simulink model "Supine_SpeedGoat_v1_final"  (R2022a)
settings: Solver=ode5  StartTime=0.0  StopTime=Inf  FixedStep=0.001  RelTol=1e-3  EnableMultiTasking=on
undefined symbols (not defined in the file): Ended, Low, Single
libraries: speedgoatlib_IO191 x5, dsparch4 x4, dspswit3 x2, slrealtimeutilitieslib x2, slrealtimeiplib x2, dspsigops x1
settings Model: SimulationMode=external  ExtModeEnableFloating=off  Creator=sjalal6  LastModifiedBy=rbme1
settings SolverCC: ConcurrentTasks=on  AlgebraicLoopSolver=TrustRegion  PositivePriorityOrder=on
settings DataIOCC: ExternalInput=waveform  LimitDataPoints=on  LoadExternalInput=on  SaveFormat=Array  SignalLoggingSaveFormat=ModelDataLogs  ReturnWorkspaceOutputs=off
settings OptimizationCC: BlockReduction=off  OptimizeBlockIOStorage=off  BufferReuse=off  ExpressionFolding=off  ExpressionDepthLimit=2147483647  LocalBlockOutputs=off
settings DebuggingCC: UnderspecifiedInitializationDetection=Classic  MergeDetectMultiDrivingBlocksExec=none  SolverPrmCheckMsg=warning  TasksWithSamePriorityMsg=none  ParameterPrecisionLossMsg=none  FcnCallInpInsideContextMsg=warning  UnconnectedInputMsg=warning  UnconnectedOutputMsg=warning  UnconnectedLineMsg=warning  StateNameClashWarn=warning  SFUnexpectedBacktrackingDiag=warning  SFNoUnconditionalDefaultTransitionDiag=warning  SFExecutionAtInitializationDiag=none  SFMachineParentedDataDiag=warning  ArithmeticOperatorsInVariantConditions=warning
settings HardwareCC: ProdBitPerLong=64  ProdLongLongMode=on  ProdHWDeviceType=Intel->x86-64 (Linux 64)
settings ModelReferenceCC: PropagateSignalLabelsOutOfModel=off
settings SFSimCC: SimUseLocalCustomCode=off  CustomCodeUndefinedFunction=UseInterfaceOnly
settings RTWCC: Description=Simulink Real-Time  SystemTargetFile=slrealtime.tlc  TemplateMakefile=slrealtime_default_tmf  RTWUseLocalCustomCode=off  Toolchain=Simulink Real-Time Toolchain  BuildConfiguration=Faster Runs  CodeExecutionProfiling=on  TargetLang=C++
settings CodeAppCC: StateflowObjectComments=on
settings ConfigComp: CovMetricSettings=dw  CovSaveCumulativeToWorkspaceVar=on  CovSaveSingleToWorkspaceVar=on  CovExternalEMLEnable=off

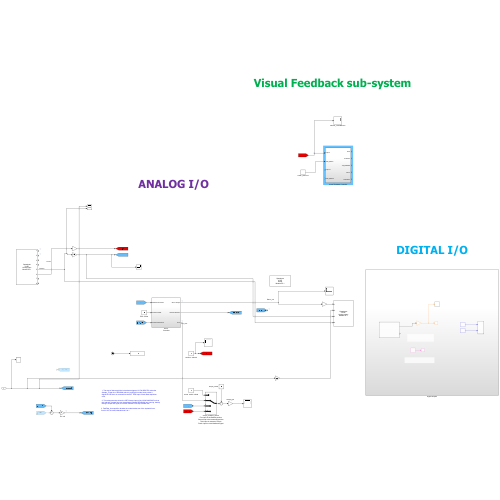
[thumbnail: Simulink's stored preview of the top-level diagram]
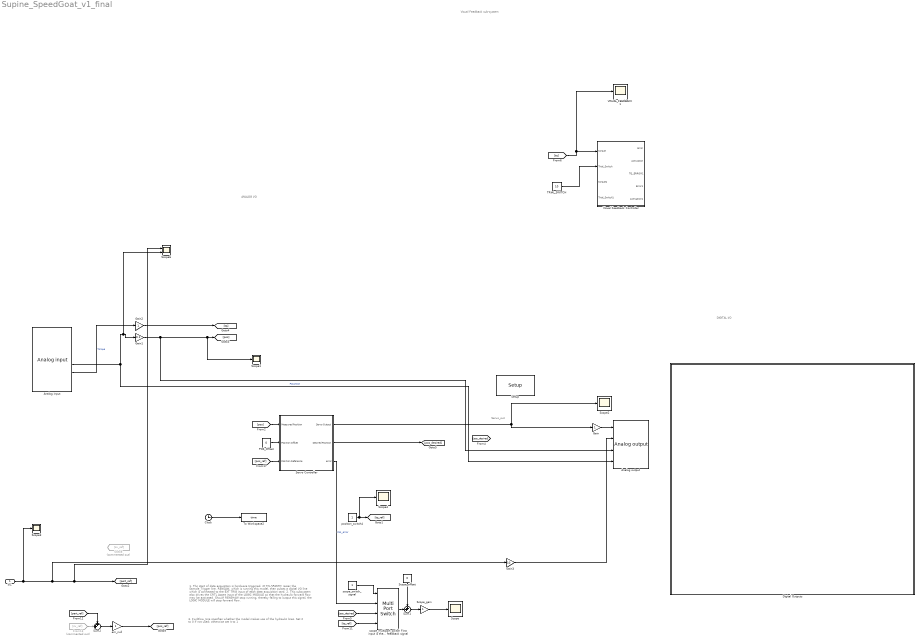
== system Supine_SpeedGoat_v1_final ==
  note: 1. The start of data acquisition is hardware triggered. 217W-SPASTIC raises the
      | Sample_Trigger line. RENSAW, which is running this model, then pulses a
      | digital I/O line which is connected to the EXT TRIG input of each data acquisition
      | card.
      |
      | 2. This subsystem also drives the CRTL Assert input of the LOGIC MODULE so that
      | the hydraulic forward flow may be activated. Should RENSHAW stop running, thereby
      | failing to output this signal, the LOGIC MODULE will stop forward flow.
  note: 3. FwdFlow_Use specifies whether the model makes use of the hydraulic lines.
      | Set it to 0 if not used; otherwise set it to 1
  note: Servo_out
  note: ANALOG I/O
  note: DIGITAL I/O
  note: Visual Feedback sub-system
  In1 : Inport
  "Analog input " : speedgoatlib_IO191/Analog input   parModuleId=1  parSampleTime=0.001  parPciSlot=-1  parAdcChannels=[1 2 3 4 5 6 7 8]  parAdcMode=2  parAdcRanges=[3 3 3 3 3 3 3 3]  parAdcRate=100000  parAdcInitValues=[0 0]  parAdcResets=[1 1]
      settings: SourceProductName=Simulink Real-Time: Speedgoat I/O Blockset
  "Analog output " : speedgoatlib_IO191/Analog output   parModuleId=1  parSampleTime=0.001  parPciSlot=-1  parDacChannels=[1 2 3 4]  parModuleType=1  parDacRanges=[4 4 4 4]  parDacInitValues=[0 0 0 0]  parDacResets=[1 1 1 1]
      settings: SourceProductName=Simulink Real-Time: Speedgoat I/O Blockset
  Clock : Clock
  Digital Outputs : Subsystem
  From13 : From  Commented=on  GotoTag=sv_ref
  Gain : Gain
  Gain1 : Gain  Gain=0.1
  Gain2 : Gain
  Gain3 : Gain  Gain=10
  Goto8 : Goto  Commented=on  GotoTag=sv_ref
  POS_Offset : Constant  Value=0
  Scope{,1..4} (5 alike) : Scope
  Scope6 : Scope  NumInputPorts=2
  Scope_gain : Gain  SaturateOnIntegerOverflow=on  OutDataTypeStr=Inherit: Same as input  ParamDataTypeStr=Inherit: Same as input
  Scope_offset : Constant  Value=0
  Servo Controller : Subsystem
  "Setup " : speedgoatlib_IO191/Setup   parModuleId=1  parPciSlot=-1  parTriggerSignal=TTL  parAdcChannels=[1 2 3 4 5 6 7 8]  parAdcRanges=[3 3 3 3 3 3 3 3]  parAdcChannel1=on  parAdcChannel2=on  parAdcChannel3=on  parAdcChannel4=on  parAdcChannel5=on  parAdcChannel6=on  parAdcChannel7=on  parAdcChannel8=on  parAdcMode=Single-Ended  parAdcRate=100000  parAdcRange11=+-10.24 V  parAdcRange21=+-24.576 V  parAdcRange12=+-10.24 V  parAdcRange22=+-24.576 V  parAdcRange13=+-10.24 V  parAdcRange23=+-24.576 V  parAdcRange14=+-10.24 V  parAdcRange24=+-24.576 V  parAdcRange15=+-10.24 V  parAdcRange25=+-24.576 V  parAdcRange16=+-10.24 V  parAdcRange26=+-24.576 V  parAdcRange17=+-10.24 V  parAdcRange27=+-24.576 V  parAdcRange18=+-10.24 V  parAdcRange28=+-24.576 V  parDacChannels=[1 2 3 4]  parDacChannel1=on  parDacChannel2=on  parDacChannel3=on  parDacChannel4=on  parDacMode=Single-Ended  parDacRanges=[4 4 4 4]  parDacInitValues=[0 0 0 0]  parDacResets=[1 1 1 1]  parDacRange1=+-10 V  parDacInitValue1=0  parDacReset1=on  parDacRange2=+-10 V  parDacInitValue2=0  parDacReset2=on  parDacRange3=+-10 V  parDacInitValue3=0  parDacReset3=on  parDacRange4=+-10 V  parDacInitValue4=0  parDacReset4=on  parDiChannels=[11 12]  parDoChannels=[1 2 3 4 5 6 7 8 9 10 13 14 15 16]  parDioFirstControl=[1 2 3 6 7 8 9]  parDioSecondControl=0  parDioChannel1=Out  parExtra1=I  parExtra2=I  parExtra3=I  parDioChannel2=Out  parDioChannel3=Out  parDioChannel4=In  parDioChannel5=In  parDioChannel6=Out  parDioChannel7=Out  parDioChannel8=Out  parDioChannel9=Out  parDoInitValues=[0 0 0 0]  parDoResets=[1 1 1 1]  parDoInitValue1=0  parDoReset1=on  parDoInitValue2=0  parDoReset2=on  parDoInitValue3=0  parDoReset3=on  parDoInitValue4=0  parDoReset4=on  parDoInitValue5=0  parDoReset5=on  parDoInitValue6=0  parDoReset6=on  parDoInitValue7=0  parDoReset7=on  parDoInitValue8=0  parDoReset8=on  parDoInitValue9=0  parDoReset9=on  parDoInitValue10=0  parDoReset10=on  parDoInitValue11=0  parDoReset11=on  parDoInitValue12=0  parDoReset12=on  parDoInitValue13=0  parDoReset13=on  parDoInitValue14=0  parDoReset14=on  parDoInitValue15=0  parDoReset15=on  parDoInitValue16=0  parDoReset16=on
      settings: SourceProductName=Simulink Real-Time: Speedgoat I/O Blockset
  Sum1 : Sum  Inputs=++|
  Sum2 : Sum  Inputs=++|
  TRIAL_SWITCH : Constant  Value=10
  To Workspace2 : ToWorkspace  VariableName=time  SampleTime=-1
  VISUAL_FEEDBACK1 : Scope
  Visual Feedback Controller : Subsystem
  em_null : Gain
  position_switch4 : Constant
  scope_multiport_switch First input is the desired position Second inpt is the measured position Third input is measured Torque Fourth input is visual feedback signal : MultiPortSwitch  SaturateOnIntegerOverflow=off  InputSameDT=off
  scope_switch_signal : Constant
  wires:
  Scope_gain/1 -> Scope/1
  Sum1/1 -> Scope_gain/1
  Scope_offset/1 -> Sum1/1
  scope_multiport_switch First input is the desired position Second inpt is the measured position Third input is measured Torque Fourth input is visual feedback signal/1 -> Sum1/2
  scope_switch_signal/1 -> scope_multiport_switch First input is the desired position Second inpt is the measured position Third input is measured Torque Fourth input is visual feedback signal/1
  POS_Offset/1 -> Servo Controller/2(Position Offset)
  [pos] -> Servo Controller/1(Measured Position)
  Servo Controller/3(error) -> scope_multiport_switch First input is the desired position Second inpt is the measured position Third input is measured Torque Fourth input is visual feedback signal/2  "Pos_error"
  Servo Controller/2(Desired Position) -> [pos_desired]
  [pos_desired] -> scope_multiport_switch First input is the desired position Second inpt is the measured position Third input is measured Torque Fourth input is visual feedback signal/3
  [tq] -> VISUAL_FEEDBACK1/1, Visual Feedback Controller/1(torque)
  [tq_ref] -> scope_multiport_switch First input is the desired position Second inpt is the measured position Third input is measured Torque Fourth input is visual feedback signal/4
  [pert_ref] -> Sum2/1
  From13/1 -> Sum2/2
  "Analog input "/6 -> Gain2/1  "Torque"
  "Analog input "/5 -> Scope6/2, Gain1/1, "Analog output "/4  "Possition"
  position_switch4/1 -> Scope4/1, [tq_ref]
  [pos_ref] -> Servo Controller/3(Position Reference)
  Servo Controller/1(Servo Output) -> Scope2/1, Gain/1
  Clock/1 -> To Workspace2/1
  Sum2/1 -> em_null/1
  Gain/1 -> "Analog output "/1
  em_null/1 -> [pos_ref]
  Gain2/1 -> [tq]
  In1/1 -> Scope3/1, Gain3/1, Scope6/1, [pert_ref]
  Gain1/1 -> "Analog output "/3, Scope1/1, [pos]
  Gain3/1 -> "Analog output "/2
  TRIAL_SWITCH/1 -> Visual Feedback Controller/2(Trial_Switch)

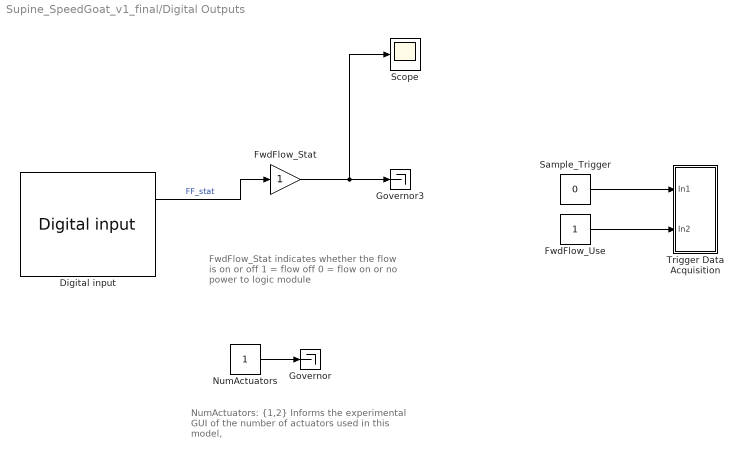
== system Supine_SpeedGoat_v1_final/Digital Outputs ==
  note: NumActuators: {1,2}
      | Informs the experimental GUI of the number
      | of actuators used in this model,
  note: FwdFlow_Stat indicates whether
      | the flow is on or off
      | 1 = flow off
      | 0 = flow on or no power to logic module
  "Digital input " : speedgoatlib_IO191/Digital input   parModuleId=1  parSampleTime=-1  parPciSlot=-1  parDiChannels=[11 12]
      settings: SourceProductName=Simulink Real-Time: Speedgoat I/O Blockset
  FwdFlow_Stat : Gain  SaturateOnIntegerOverflow=on  OutDataTypeStr=Inherit: Same as input  ParamDataTypeStr=Inherit: Same as input
  FwdFlow_Use : Constant
  Governor : Terminator
  Governor3 : Terminator
  NumActuators : Constant
  Sample_Trigger : Constant  Value=0
  Scope : Scope
  Trigger Data Acquisition : Subsystem
  wires:
  FwdFlow_Use/1 -> Trigger Data Acquisition/2(In2)
  NumActuators/1 -> Governor/1
  FwdFlow_Stat/1 -> Scope/1, Governor3/1
  "Digital input "/1 -> FwdFlow_Stat/1  "FF_stat"
  Sample_Trigger/1 -> Trigger Data Acquisition/1(In1)

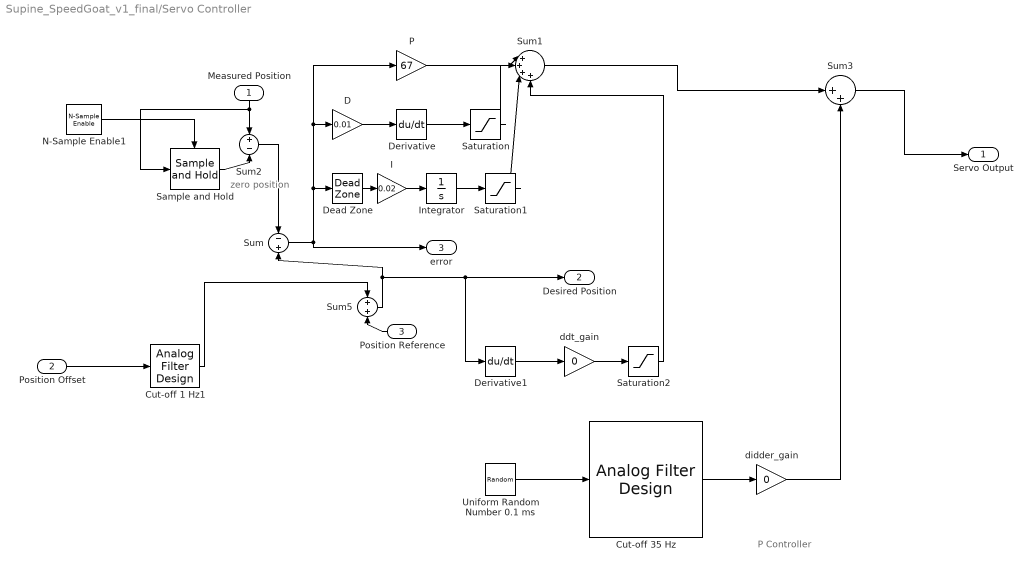
== system Supine_SpeedGoat_v1_final/Servo Controller ==
  note: zero
      | position
  note: P Controller
  Measured Position : Inport
  Position Offset : Inport  Port=2
  Position Reference : Inport  Port=3
  Cut-off 1 Hz1 : dsparch4/Analog Filter Design  method=Bessel  filttype=Lowpass  N=2  Wlo=2*1*pi  Whi=80  Rp=2  Rs=40
  Cut-off 35 Hz : dsparch4/Analog Filter Design  method=Bessel  filttype=Highpass  N=5  Wlo=2*pi*40  Whi=80  Rp=0.01  Rs=40
  D : Gain  Gain=0.01  SaturateOnIntegerOverflow=on  OutDataTypeStr=Inherit: Same as input  ParamDataTypeStr=Inherit: Same as input
  Dead Zone : DeadZone  LowerValue=-0.01  UpperValue=0.01
  Derivative : Derivative
  Derivative1 : Derivative
  I : Gain  Gain=0.02  SaturateOnIntegerOverflow=on  OutDataTypeStr=Inherit: Same as input  ParamDataTypeStr=Inherit: Same as input
  Integrator : Integrator  LimitOutput=on  UpperSaturationLimit=1  LowerSaturationLimit=-1
  N-Sample Enable1 : dspswit3/N-Sample Enable  N=100  ActiveLevel=Low (0)  reset=off  TriggerType=Rising edge  Ts=0.001  DataType=Logical
      settings: SourceProductBaseCode=DS
  P : Gain  Gain=67  SaturateOnIntegerOverflow=on  OutDataTypeStr=Inherit: Same as input  ParamDataTypeStr=Inherit: Same as input
  Sample and Hold : dspsigops/Sample and Hold  trig=Falling edge  initCond=0  latchinput=off
  Saturation : Saturate
  Saturation1 : Saturate  UpperLimit=1  LowerLimit=-1
  Saturation2 : Saturate  UpperLimit=1  LowerLimit=-1
  Sum : Sum  Inputs=-+  InputSameDT=on  SaturateOnIntegerOverflow=on  OutDataTypeStr=Inherit: Same as first input
  Sum1 : Sum  Inputs=|++++  InputSameDT=on  SaturateOnIntegerOverflow=on  OutDataTypeStr=Inherit: Same as first input
  Sum2 : Sum  Inputs=+|-  InputSameDT=on  SaturateOnIntegerOverflow=on  OutDataTypeStr=Inherit: Same as first input
  Sum3 : Sum  Inputs=|++  InputSameDT=on  SaturateOnIntegerOverflow=on  OutDataTypeStr=Inherit: Same as first input
  Sum5 : Sum  InputSameDT=on  SaturateOnIntegerOverflow=on  OutDataTypeStr=Inherit: Same as first input
  Uniform Random Number 0.1 ms : UniformRandomNumber  SampleTime=0.001
  ddt_gain : Gain  Gain=0  SaturateOnIntegerOverflow=on  OutDataTypeStr=Inherit: Same as input  ParamDataTypeStr=Inherit: Same as input
  didder_gain : Gain  Gain=0  SaturateOnIntegerOverflow=on  OutDataTypeStr=Inherit: Same as input  ParamDataTypeStr=Inherit: Same as input
  Servo Output : Outport
  Desired Position : Outport  Port=2
  error : Outport  Port=3
  wires:
  Sum5/1 -> Sum/2, Derivative1/1, Desired Position/1
  Cut-off 1 Hz1/1 -> Sum5/1
  Sum2/1 -> Sum/1
  N-Sample Enable1/1 -> Sample and Hold/Trigger
  Sample and Hold/1 -> Sum2/2
  Sum/1 -> Dead Zone/1, D/1, P/1, error/1
  Measured Position/1 -> Sum2/1, Sample and Hold/1
  Position Reference/1 -> Sum5/2
  Position Offset/1 -> Cut-off 1 Hz1/1
  D/1 -> Derivative/1
  P/1 -> Sum1/1
  Derivative/1 -> Saturation/1
  Saturation/1 -> Sum1/2
  I/1 -> Integrator/1
  Integrator/1 -> Saturation1/1
  Saturation1/1 -> Sum1/3
  Dead Zone/1 -> I/1
  Derivative1/1 -> ddt_gain/1
  ddt_gain/1 -> Saturation2/1
  Saturation2/1 -> Sum1/4
  Sum1/1 -> Sum3/1
  Sum3/1 -> Servo Output/1
  Cut-off 35 Hz/1 -> didder_gain/1
  Uniform Random Number 0.1 ms/1 -> Cut-off 35 Hz/1
  didder_gain/1 -> Sum3/2

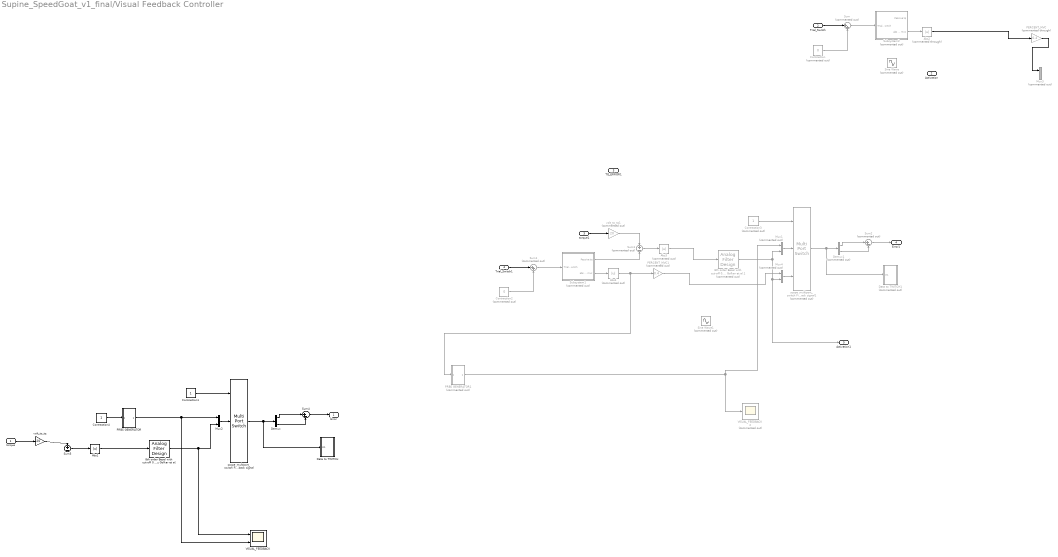
== system Supine_SpeedGoat_v1_final/Visual Feedback Controller ==
  torque : Inport
  Trial_Switch : Inport  Port=2
  torque1 : Inport  Port=3
  Trial_Switch1 : Inport  Port=4
  8th order Besel with cut-off 0.7 Hz Golkar et al. : dsparch4/Analog Filter Design  method=Bessel  filttype=Lowpass  N=8  Wlo=2*pi*20  Whi=80  Rp=2  Rs=40
  8th order Besel with cut-off 0.7 Hz Golkar et al.1 : dsparch4/Analog Filter Design  Commented=on  method=Bessel  filttype=Lowpass  N=8  Wlo=2*pi*20  Whi=80  Rp=2  Rs=40
  Abs1 : Abs  SaturateOnIntegerOverflow=off
  Abs2 : Abs  Commented=through  SaturateOnIntegerOverflow=off
  Abs3 : Abs  Commented=on  SaturateOnIntegerOverflow=off
  Abs4 : Abs  Commented=on  SaturateOnIntegerOverflow=off
  Contraction : Constant  Commented=on  Value=0
  Contraction1 : Constant
  Contraction2 : Constant  Commented=on  Value=0
  Contraction3 : Constant  Commented=on
  Contraction4 : Constant
  Data to TWITCH : Subsystem
  Data to TWITCH1 : Subsystem  Commented=on
  Demux : Demux  Outputs=2
  Demux1 : Demux  Commented=on  Outputs=2
  Mux1 : Mux  Commented=on  Inputs=2
  Mux2 : Mux  Inputs=2
  Mux3 : Mux  Commented=on  Inputs=2
  Mux4 : Mux  Commented=on  Inputs=2
  PERCENT_MVC : Gain  Commented=through  Gain=0.4  SaturateOnIntegerOverflow=on  OutDataTypeStr=Inherit: Same as input  ParamDataTypeStr=Inherit: Same as input
  PERCENT_MVC1 : Gain  Commented=on  Gain=0.4  SaturateOnIntegerOverflow=on  OutDataTypeStr=Inherit: Same as input  ParamDataTypeStr=Inherit: Same as input
  PRBS GENERATOR : Subsystem
  PRBS GENERATOR1 : Subsystem  Commented=on
  Sine Wave : Sin  Commented=on  Amplitude=5  Bias=5  Frequency=4*pi*(1/20)  Phase=-pi/2  SampleTime=0
  Sine Wave1 : Sin  Commented=on  Amplitude=5  Bias=5  Frequency=4*pi*(1/20)  Phase=-pi/2  SampleTime=0
  Subsystem1 : Subsystem  Commented=on
  Subsystem2 : Subsystem  Commented=on
  Sum : Sum  Commented=on  Inputs=|++
  Sum1 : Sum  Commented=on  Inputs=|++
  Sum2 : Sum  Commented=on  Inputs=|+-  InputSameDT=on  SaturateOnIntegerOverflow=on  OutDataTypeStr=Inherit: Same as first input
  Sum3 : Sum  Commented=on  Inputs=+-  InputSameDT=on  SaturateOnIntegerOverflow=on  OutDataTypeStr=Inherit: Same as first input
  Sum4 : Sum  Inputs=|+-  InputSameDT=on  SaturateOnIntegerOverflow=on  OutDataTypeStr=Inherit: Same as first input
  Sum5 : Sum  Inputs=+-  InputSameDT=on  SaturateOnIntegerOverflow=on  OutDataTypeStr=Inherit: Same as first input
  VISUAL_FEEDBACK : Scope  NumInputPorts=2
  VISUAL_FEEDBACK2 : Scope  Commented=on
  scope_multiport_switch First input is the desired position Second inpt is the measured position Third input is measured Torque Fourth input is visual feedback signal : MultiPortSwitch  Inputs=2  SaturateOnIntegerOverflow=off  InputSameDT=off
  scope_multiport_switch First input is the desired position Second inpt is the measured position Third input is measured Torque Fourth input is visual feedback signal1 : MultiPortSwitch  Commented=on  Inputs=2  SaturateOnIntegerOverflow=off  InputSameDT=off
  volt_to_tq : Gain  Gain=20  SaturateOnIntegerOverflow=on  OutDataTypeStr=Inherit: Same as input  ParamDataTypeStr=Inherit: Same as input
  volt_to_tq1 : Gain  Commented=on  Gain=20  SaturateOnIntegerOverflow=on  OutDataTypeStr=Inherit: Same as input  ParamDataTypeStr=Inherit: Same as input
  Error : Outport
  Activation : Outport  Port=2
  TQ_ERROR1 : Outport  Port=3
  Error1 : Outport  Port=4
  Activation1 : Outport  Port=5
  wires:
  torque/1 -> volt_to_tq/1
  volt_to_tq/1 -> Sum5/1
  Subsystem2/2(abs 0.15 mvc) -> Abs2/1
  Sum5/1 -> Abs1/1
  Trial_Switch/1 -> Sum/1
  Contraction/1 -> Sum/2
  Sum/1 -> Subsystem2/1(Trial_Switch)
  Mux2/1 -> scope_multiport_switch First input is the desired position Second inpt is the measured position Third input is measured Torque Fourth input is visual feedback signal/2
  Sum4/1 -> Error/1
  Demux/1 -> Sum4/1
  scope_multiport_switch First input is the desired position Second inpt is the measured position Third input is measured Torque Fourth input is visual feedback signal/1 -> Data to TWITCH/1(In1), Demux/1
  8th order Besel with cut-off 0.7 Hz Golkar et al./1 -> VISUAL_FEEDBACK/1, Mux2/2
  Demux/2 -> Sum4/2
  Contraction1/1 -> scope_multiport_switch First input is the desired position Second inpt is the measured position Third input is measured Torque Fourth input is visual feedback signal/1
  Abs1/1 -> 8th order Besel with cut-off 0.7 Hz Golkar et al./1
  PERCENT_MVC/1 -> Mux3/1
  PRBS GENERATOR/1(Out1) -> VISUAL_FEEDBACK/2, Mux2/1
  Abs2/1 -> PERCENT_MVC/1
  Contraction3/1 -> scope_multiport_switch First input is the desired position Second inpt is the measured position Third input is measured Torque Fourth input is visual feedback signal1/1
  Mux1/1 -> scope_multiport_switch First input is the desired position Second inpt is the measured position Third input is measured Torque Fourth input is visual feedback signal1/2
  Sum3/1 -> Abs3/1
  8th order Besel with cut-off 0.7 Hz Golkar et al.1/1 -> Activation1/1, Mux4/2, Mux1/2
  Subsystem1/1(Passive tq) -> Sum3/2
  Contraction2/1 -> Sum1/2
  Trial_Switch1/1 -> Sum1/1
  Mux4/1 -> scope_multiport_switch First input is the desired position Second inpt is the measured position Third input is measured Torque Fourth input is visual feedback signal1/3
  Sum2/1 -> Error1/1
  Demux1/1 -> Sum2/1
  scope_multiport_switch First input is the desired position Second inpt is the measured position Third input is measured Torque Fourth input is visual feedback signal1/1 -> Data to TWITCH1/1(In1), Demux1/1
  volt_to_tq1/1 -> Sum3/1
  torque1/1 -> volt_to_tq1/1
  Demux1/2 -> Sum2/2
  Abs4/1 -> PRBS GENERATOR1/1(abs mvc), PERCENT_MVC1/1
  Sum1/1 -> Subsystem1/1(Trial_Switch)
  PRBS GENERATOR1/1(Out1) -> Mux1/1, VISUAL_FEEDBACK2/1
  Abs3/1 -> 8th order Besel with cut-off 0.7 Hz Golkar et al.1/1
  PERCENT_MVC1/1 -> Mux4/1
  Subsystem1/2(abs 0.15 mvc) -> Abs4/1
  Contraction4/1 -> PRBS GENERATOR/1(abs mvc)

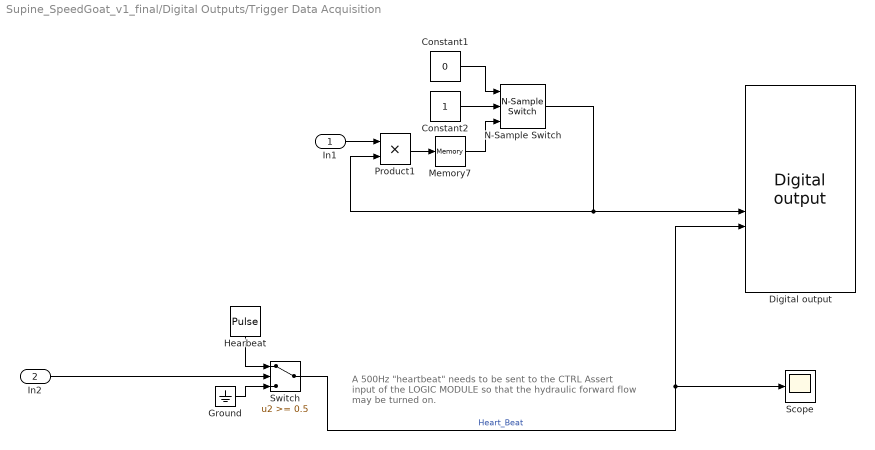
== system Supine_SpeedGoat_v1_final/Digital Outputs/Trigger Data Acquisition ==
  note: A 500Hz "heartbeat" needs to be sent to the CTRL Assert
      | input of the LOGIC MODULE so that the hydraulic forward
      | flow may be turned on.
  In1 : Inport
  In2 : Inport  Port=2
  Constant1 : Constant  Value=0
  Constant2 : Constant
  "Digital output " : speedgoatlib_IO191/Digital output   parModuleId=1  parSampleTime=0.001  parPciSlot=-1  parDoChannels=[1 2 3 4 5 6 7 8 9 10 13 14 15 16]  parDoInitValues=[0 0 0 0 0 0 0 0 0 0 0 0 0 0]  parDoResets=[1 1 1 1 1 1 1 1 1 1 1 1 1 1]
      settings: SourceProductName=Simulink Real-Time: Speedgoat I/O Blockset
  Ground : Ground
  Hearbeat : DiscretePulseGenerator  PulseType=Time based  Period=1/500  PulseWidth=50  SampleTime=0.001
  Memory7 : Memory  InheritSampleTime=on
  N-Sample Switch : dspswit3/N-Sample Switch  N=1000  reset=on  TriggerType=Rising edge  Ts=0.001
      settings: SourceProductBaseCode=DS
  Product1 : Product  RndMeth=Zero
  Scope : Scope
  Switch : Switch  Threshold=0.5  SaturateOnIntegerOverflow=off  InputSameDT=off
  wires:
  Constant1/1 -> N-Sample Switch/1
  Constant2/1 -> N-Sample Switch/2
  N-Sample Switch/1 -> "Digital output "/9, Product1/2
  Product1/1 -> Memory7/1
  Memory7/1 -> N-Sample Switch/3
  In1/1 -> Product1/1
  Switch/1 -> Scope/1, "Digital output "/10  "Heart_Beat"
  Hearbeat/1 -> Switch/1
  In2/1 -> Switch/2
  Ground/1 -> Switch/3

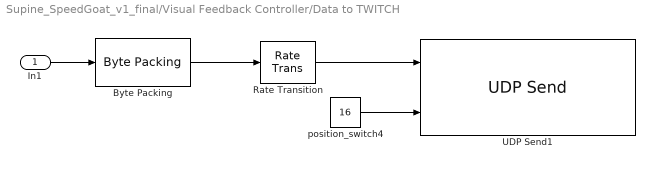
== system Supine_SpeedGoat_v1_final/Visual Feedback Controller/Data to TWITCH ==
  In1 : Inport
  Byte Packing : slrealtimeutilitieslib/Byte Packing  MaskPackedDataType=uint8  MaskUnpackedDataTypes={'double'}  MaskAlignment=1
  Rate Transition : RateTransition
  UDP Send1 : slrealtimeiplib/UDP Send  useHostTargetConn=off  toAddress='10.68.3.239'  toPort=5005  sampleTime=0.02  enableMessage=off  ipAddress=10.68.3.237  localPort=5005
      settings: SourceProductBaseCode=XP
  position_switch4 : Constant  Value=16
  wires:
  Byte Packing/1 -> Rate Transition/1
  Rate Transition/1 -> UDP Send1/1
  In1/1 -> Byte Packing/1
  position_switch4/1 -> UDP Send1/2

== system Supine_SpeedGoat_v1_final/Visual Feedback Controller/Data to TWITCH1 ==
  In1 : Inport
  Byte Packing : slrealtimeutilitieslib/Byte Packing  MaskPackedDataType=uint8  MaskUnpackedDataTypes={'double'}  MaskAlignment=1
  Rate Transition : RateTransition
  UDP Send1 : slrealtimeiplib/UDP Send  useHostTargetConn=off  toAddress='10.68.3.239'  toPort=5005  sampleTime=0.02  enableMessage=off  ipAddress=10.68.3.237  localPort=5005
      settings: SourceProductBaseCode=XP
  position_switch4 : Constant  Value=16
  wires:
  Byte Packing/1 -> Rate Transition/1
  Rate Transition/1 -> UDP Send1/1
  In1/1 -> Byte Packing/1
  position_switch4/1 -> UDP Send1/2

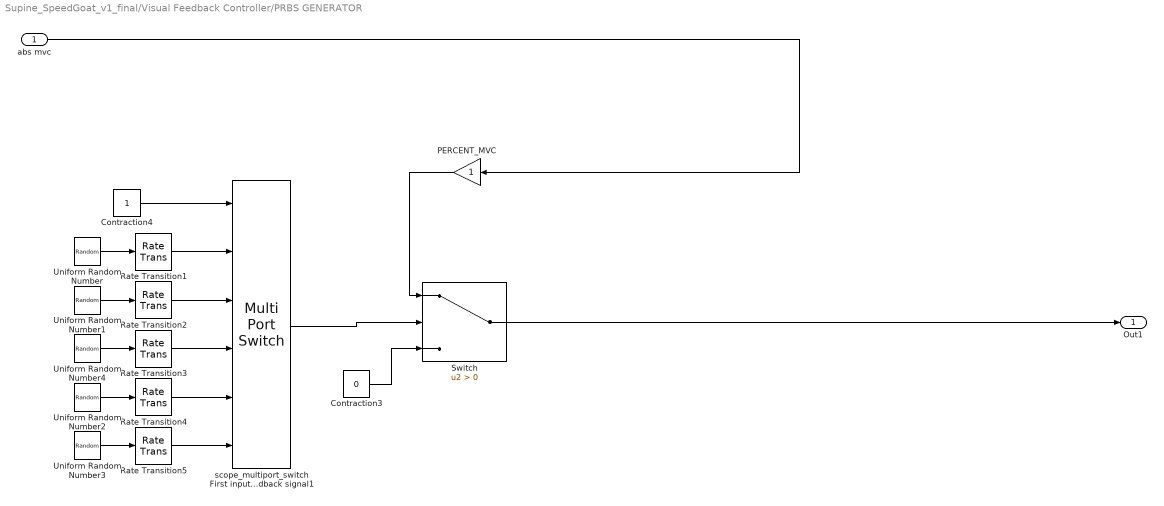
== system Supine_SpeedGoat_v1_final/Visual Feedback Controller/PRBS GENERATOR ==
  abs mvc : Inport
  Contraction3 : Constant  Value=0
  Contraction4 : Constant
  PERCENT_MVC : Gain  SaturateOnIntegerOverflow=on  OutDataTypeStr=Inherit: Same as input  ParamDataTypeStr=Inherit: Same as input
  Rate Transition{1..5} (5 alike) : RateTransition  OutPortSampleTime=0
  Switch : Switch  Criteria=u2 > Threshold  SaturateOnIntegerOverflow=off  InputSameDT=off
  Uniform Random Number : UniformRandomNumber  SampleTime=0.2
  Uniform Random Number1 : UniformRandomNumber  SampleTime=0.5
  Uniform Random Number2 : UniformRandomNumber  SampleTime=2
  Uniform Random Number3 : UniformRandomNumber  SampleTime=4
  Uniform Random Number4 : UniformRandomNumber  SampleTime=1
  scope_multiport_switch First input is the desired position Second inpt is the measured position Third input is measured Torque Fourth input is visual feedback signal1 : MultiPortSwitch  Inputs=5  SaturateOnIntegerOverflow=off  InputSameDT=off
  Out1 : Outport
  wires:
  Rate Transition2/1 -> scope_multiport_switch First input is the desired position Second inpt is the measured position Third input is measured Torque Fourth input is visual feedback signal1/3
  Uniform Random Number2/1 -> Rate Transition4/1
  Uniform Random Number1/1 -> Rate Transition2/1
  Uniform Random Number3/1 -> Rate Transition5/1
  Rate Transition4/1 -> scope_multiport_switch First input is the desired position Second inpt is the measured position Third input is measured Torque Fourth input is visual feedback signal1/5
  Rate Transition1/1 -> scope_multiport_switch First input is the desired position Second inpt is the measured position Third input is measured Torque Fourth input is visual feedback signal1/2
  Rate Transition5/1 -> scope_multiport_switch First input is the desired position Second inpt is the measured position Third input is measured Torque Fourth input is visual feedback signal1/6
  Uniform Random Number/1 -> Rate Transition1/1
  Contraction3/1 -> Switch/3
  Contraction4/1 -> scope_multiport_switch First input is the desired position Second inpt is the measured position Third input is measured Torque Fourth input is visual feedback signal1/1
  Uniform Random Number4/1 -> Rate Transition3/1
  Rate Transition3/1 -> scope_multiport_switch First input is the desired position Second inpt is the measured position Third input is measured Torque Fourth input is visual feedback signal1/4
  scope_multiport_switch First input is the desired position Second inpt is the measured position Third input is measured Torque Fourth input is visual feedback signal1/1 -> Switch/2
  Switch/1 -> Out1/1
  abs mvc/1 -> PERCENT_MVC/1
  PERCENT_MVC/1 -> Switch/1

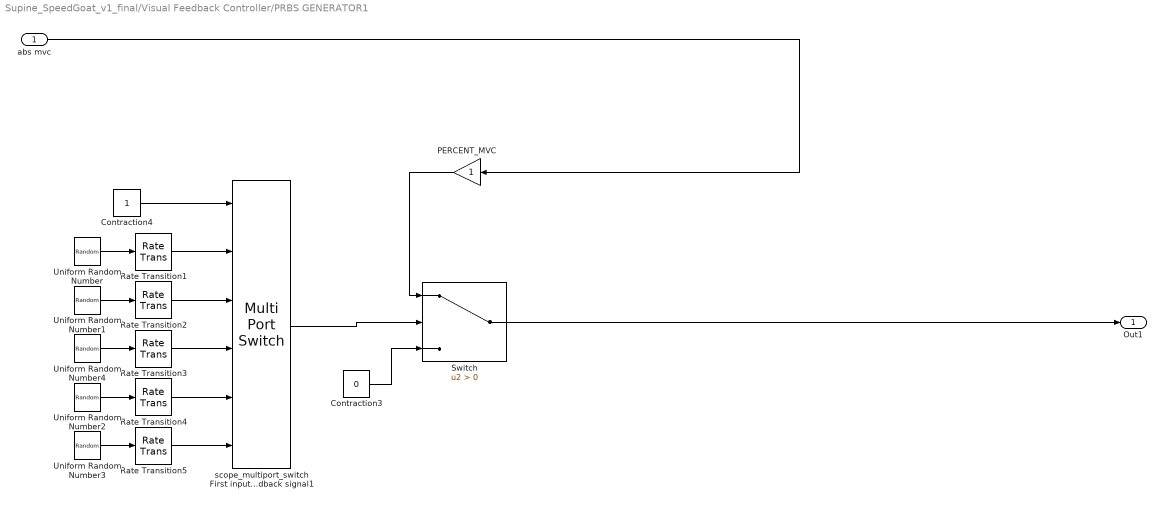
== system Supine_SpeedGoat_v1_final/Visual Feedback Controller/PRBS GENERATOR1 ==
  abs mvc : Inport
  Contraction3 : Constant  Value=0
  Contraction4 : Constant
  PERCENT_MVC : Gain  SaturateOnIntegerOverflow=on  OutDataTypeStr=Inherit: Same as input  ParamDataTypeStr=Inherit: Same as input
  Rate Transition{1..5} (5 alike) : RateTransition  OutPortSampleTime=0
  Switch : Switch  Criteria=u2 > Threshold  SaturateOnIntegerOverflow=off  InputSameDT=off
  Uniform Random Number : UniformRandomNumber  SampleTime=0.2
  Uniform Random Number1 : UniformRandomNumber  SampleTime=0.5
  Uniform Random Number2 : UniformRandomNumber  SampleTime=2
  Uniform Random Number3 : UniformRandomNumber  SampleTime=4
  Uniform Random Number4 : UniformRandomNumber  SampleTime=1
  scope_multiport_switch First input is the desired position Second inpt is the measured position Third input is measured Torque Fourth input is visual feedback signal1 : MultiPortSwitch  Inputs=5  SaturateOnIntegerOverflow=off  InputSameDT=off
  Out1 : Outport
  wires:
  Rate Transition2/1 -> scope_multiport_switch First input is the desired position Second inpt is the measured position Third input is measured Torque Fourth input is visual feedback signal1/3
  Uniform Random Number2/1 -> Rate Transition4/1
  Uniform Random Number1/1 -> Rate Transition2/1
  Uniform Random Number3/1 -> Rate Transition5/1
  Rate Transition4/1 -> scope_multiport_switch First input is the desired position Second inpt is the measured position Third input is measured Torque Fourth input is visual feedback signal1/5
  Rate Transition1/1 -> scope_multiport_switch First input is the desired position Second inpt is the measured position Third input is measured Torque Fourth input is visual feedback signal1/2
  Rate Transition5/1 -> scope_multiport_switch First input is the desired position Second inpt is the measured position Third input is measured Torque Fourth input is visual feedback signal1/6
  Uniform Random Number/1 -> Rate Transition1/1
  Contraction3/1 -> Switch/3
  Contraction4/1 -> scope_multiport_switch First input is the desired position Second inpt is the measured position Third input is measured Torque Fourth input is visual feedback signal1/1
  Uniform Random Number4/1 -> Rate Transition3/1
  Rate Transition3/1 -> scope_multiport_switch First input is the desired position Second inpt is the measured position Third input is measured Torque Fourth input is visual feedback signal1/4
  scope_multiport_switch First input is the desired position Second inpt is the measured position Third input is measured Torque Fourth input is visual feedback signal1/1 -> Switch/2
  Switch/1 -> Out1/1
  abs mvc/1 -> PERCENT_MVC/1
  PERCENT_MVC/1 -> Switch/1

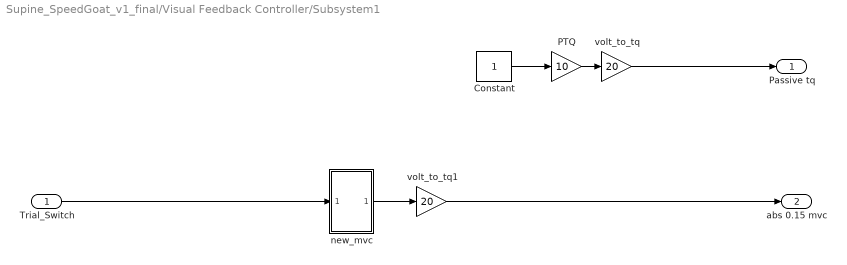
== system Supine_SpeedGoat_v1_final/Visual Feedback Controller/Subsystem1 ==
  Trial_Switch : Inport
  Constant : Constant
  PTQ : Gain  Gain=10  SaturateOnIntegerOverflow=on  OutDataTypeStr=Inherit: Same as input  ParamDataTypeStr=Inherit: Same as input
  new_mvc : Subsystem
  volt_to_tq : Gain  Gain=20  SaturateOnIntegerOverflow=on  OutDataTypeStr=Inherit: Same as input  ParamDataTypeStr=Inherit: Same as input
  volt_to_tq1 : Gain  Gain=20  SaturateOnIntegerOverflow=on  OutDataTypeStr=Inherit: Same as input  ParamDataTypeStr=Inherit: Same as input
  Passive tq : Outport
  abs 0.15 mvc : Outport  Port=2
  wires:
  Trial_Switch/1 -> new_mvc/1(In1)
  volt_to_tq1/1 -> abs 0.15 mvc/1
  new_mvc/1(Out1) -> volt_to_tq1/1
  Constant/1 -> PTQ/1
  PTQ/1 -> volt_to_tq/1
  volt_to_tq/1 -> Passive tq/1

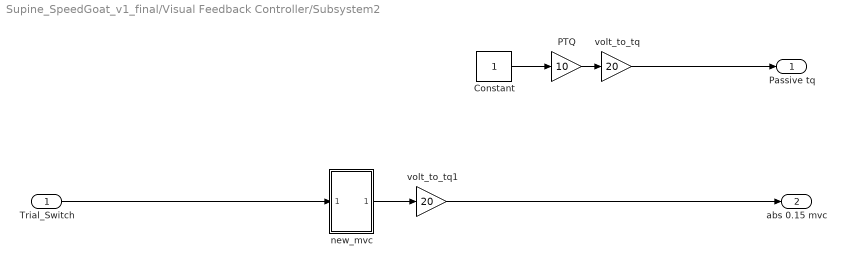
== system Supine_SpeedGoat_v1_final/Visual Feedback Controller/Subsystem2 ==
  Trial_Switch : Inport
  Constant : Constant
  PTQ : Gain  Gain=10  SaturateOnIntegerOverflow=on  OutDataTypeStr=Inherit: Same as input  ParamDataTypeStr=Inherit: Same as input
  new_mvc : Subsystem
  volt_to_tq : Gain  Gain=20  SaturateOnIntegerOverflow=on  OutDataTypeStr=Inherit: Same as input  ParamDataTypeStr=Inherit: Same as input
  volt_to_tq1 : Gain  Gain=20  SaturateOnIntegerOverflow=on  OutDataTypeStr=Inherit: Same as input  ParamDataTypeStr=Inherit: Same as input
  Passive tq : Outport
  abs 0.15 mvc : Outport  Port=2
  wires:
  Trial_Switch/1 -> new_mvc/1(In1)
  volt_to_tq1/1 -> abs 0.15 mvc/1
  new_mvc/1(Out1) -> volt_to_tq1/1
  Constant/1 -> PTQ/1
  PTQ/1 -> volt_to_tq/1
  volt_to_tq/1 -> Passive tq/1

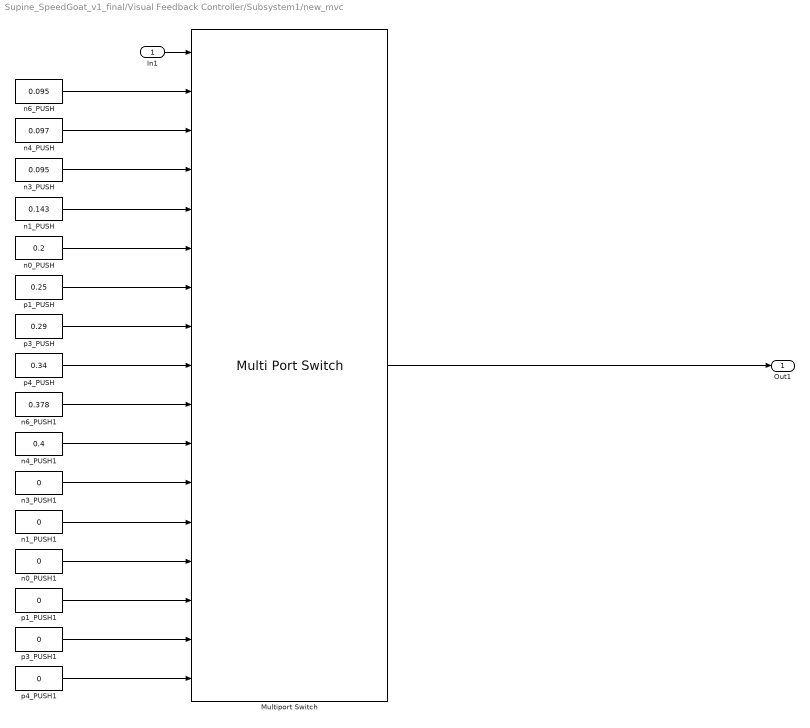
== system Supine_SpeedGoat_v1_final/Visual Feedback Controller/Subsystem1/new_mvc ==
  In1 : Inport
  Multiport Switch : MultiPortSwitch  Inputs=16  SaturateOnIntegerOverflow=off  InputSameDT=off
  n0_PUSH : Constant  Value=0.2
  n0_PUSH1 : Constant  Value=0
  n1_PUSH : Constant  Value=0.143
  n1_PUSH1 : Constant  Value=0
  n3_PUSH : Constant  Value=0.095
  n3_PUSH1 : Constant  Value=0
  n4_PUSH : Constant  Value=0.097
  n4_PUSH1 : Constant  Value=0.4
  n6_PUSH : Constant  Value=0.095
  n6_PUSH1 : Constant  Value=0.378
  p1_PUSH : Constant  Value=0.25
  p1_PUSH1 : Constant  Value=0
  p3_PUSH : Constant  Value=0.29
  p3_PUSH1 : Constant  Value=0
  p4_PUSH : Constant  Value=0.34
  p4_PUSH1 : Constant  Value=0
  Out1 : Outport
  wires:
  n6_PUSH/1 -> Multiport Switch/2
  n4_PUSH/1 -> Multiport Switch/3
  n3_PUSH/1 -> Multiport Switch/4
  n1_PUSH/1 -> Multiport Switch/5
  n0_PUSH/1 -> Multiport Switch/6
  p1_PUSH/1 -> Multiport Switch/7
  p3_PUSH/1 -> Multiport Switch/8
  p4_PUSH/1 -> Multiport Switch/9
  In1/1 -> Multiport Switch/1
  Multiport Switch/1 -> Out1/1
  n3_PUSH1/1 -> Multiport Switch/12
  n4_PUSH1/1 -> Multiport Switch/11
  n0_PUSH1/1 -> Multiport Switch/14
  p3_PUSH1/1 -> Multiport Switch/16
  n1_PUSH1/1 -> Multiport Switch/13
  p4_PUSH1/1 -> Multiport Switch/17
  n6_PUSH1/1 -> Multiport Switch/10
  p1_PUSH1/1 -> Multiport Switch/15

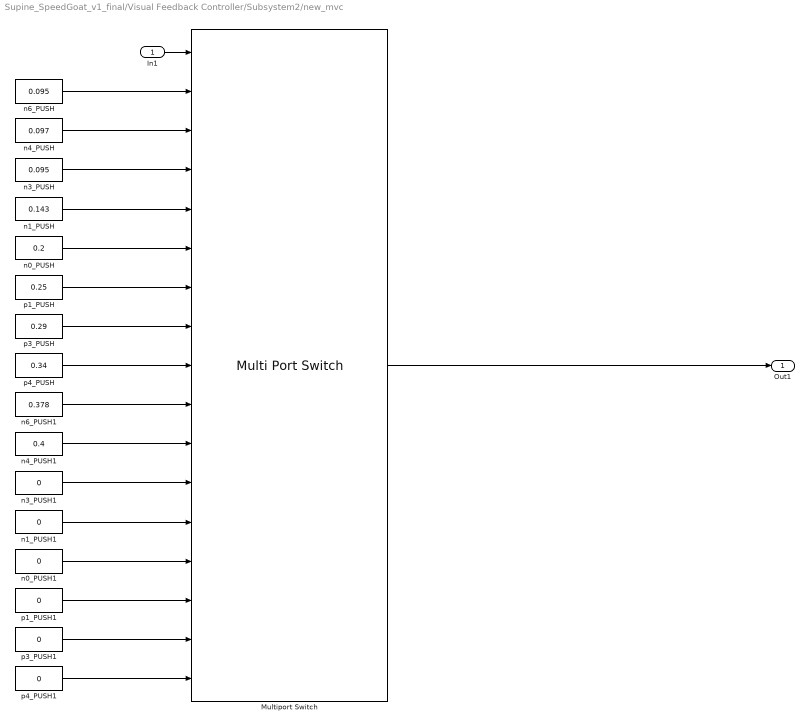
== system Supine_SpeedGoat_v1_final/Visual Feedback Controller/Subsystem2/new_mvc ==
  In1 : Inport
  Multiport Switch : MultiPortSwitch  Inputs=16  SaturateOnIntegerOverflow=off  InputSameDT=off
  n0_PUSH : Constant  Value=0.2
  n0_PUSH1 : Constant  Value=0
  n1_PUSH : Constant  Value=0.143
  n1_PUSH1 : Constant  Value=0
  n3_PUSH : Constant  Value=0.095
  n3_PUSH1 : Constant  Value=0
  n4_PUSH : Constant  Value=0.097
  n4_PUSH1 : Constant  Value=0.4
  n6_PUSH : Constant  Value=0.095
  n6_PUSH1 : Constant  Value=0.378
  p1_PUSH : Constant  Value=0.25
  p1_PUSH1 : Constant  Value=0
  p3_PUSH : Constant  Value=0.29
  p3_PUSH1 : Constant  Value=0
  p4_PUSH : Constant  Value=0.34
  p4_PUSH1 : Constant  Value=0
  Out1 : Outport
  wires:
  n6_PUSH/1 -> Multiport Switch/2
  n4_PUSH/1 -> Multiport Switch/3
  n3_PUSH/1 -> Multiport Switch/4
  n1_PUSH/1 -> Multiport Switch/5
  n0_PUSH/1 -> Multiport Switch/6
  p1_PUSH/1 -> Multiport Switch/7
  p3_PUSH/1 -> Multiport Switch/8
  p4_PUSH/1 -> Multiport Switch/9
  In1/1 -> Multiport Switch/1
  Multiport Switch/1 -> Out1/1
  n3_PUSH1/1 -> Multiport Switch/12
  n4_PUSH1/1 -> Multiport Switch/11
  n0_PUSH1/1 -> Multiport Switch/14
  p3_PUSH1/1 -> Multiport Switch/16
  n1_PUSH1/1 -> Multiport Switch/13
  p4_PUSH1/1 -> Multiport Switch/17
  n6_PUSH1/1 -> Multiport Switch/10
  p1_PUSH1/1 -> Multiport Switch/15
